simulink model "Track_green_simulation"  (R2021b)
settings: Solver=FixedStepDiscrete  StartTime=0.0  StopTime=inf  RelTol=1e-3  EnableMultiTasking=on
libraries: visionsinks x2, visiontextngfix x1, dspvision x1, simulink x1
settings Model: SimulationMode=external  ExtModeTrigDuration=100  Creator=edelaher  LastModifiedBy=litani
settings SolverCC: AlgebraicLoopSolver=TrustRegion  PositivePriorityOrder=on  AutoInsertRateTranBlk=on
settings DataIOCC: LimitDataPoints=on  SaveFormat=Array  ReturnWorkspaceOutputs=off
settings OptimizationCC: DefaultParameterBehavior=Inlined  MaxStackSize=64  EfficientTunableParamExpr=on
settings DebuggingCC: UnderspecifiedInitializationDetection=Classic  MergeDetectMultiDrivingBlocksExec=none  ParameterTunabilityLossMsg=error  AllowSymbolicDim=off  SFUnexpectedBacktrackingDiag=warning  SFNoUnconditionalDefaultTransitionDiag=warning  SFExecutionAtInitializationDiag=none  SFMachineParentedDataDiag=warning  ArithmeticOperatorsInVariantConditions=warning
settings HardwareCC: ProdBitPerPointer=32  ProdBitPerSizeT=32  ProdBitPerPtrDiffT=32  ProdLargestAtomicInteger=Long  ProdLargestAtomicFloat=Double  ProdWordSize=32  ProdHWDeviceType=ARM Compatible->ARM Cortex  UseEmbeddedCoderFeatures=off
settings ModelReferenceCC: PropagateSignalLabelsOutOfModel=off
settings SFSimCC: SimUseLocalCustomCode=off  MATLABDynamicMemAlloc=off  CustomCodeUndefinedFunction=UseInterfaceOnly
settings RTWCC: Description=Embedded Coder  SystemTargetFile=ert.tlc  TemplateMakefile=ert_default_tmf  GenerateReport=on  RTWVerbose=off  RTWUseLocalCustomCode=off  Toolchain=GNU GCC Embedded Linux  IncludeHyperlinkInReport=on  LaunchReport=on  GenerateTraceInfo=on  GenerateTraceReport=on  GenerateTraceReportSl=on  GenerateTraceReportSf=on  GenerateTraceReportEml=on
settings CodeAppCC: ForceParamTrailComments=on  IgnoreCustomStorageClasses=off  OperatorAnnotations=on  SimulinkDataObjDesc=on  SFDataObjDesc=on  MATLABFcnDesc=on  InsertBlockDesc=on  StateflowObjectComments=on  MATLABSourceComments=on
settings ERTTargetCC: MultiwordLength=2048  SupportNonInlinedSFcns=on  SupportVariableSizeSignals=on  ERTCustomFileTemplate=example_file_process.tlc
settings ConfigComp: CovMetricSettings=dw  CovSaveCumulativeToWorkspaceVar=on  CovSaveSingleToWorkspaceVar=on  CovExternalEMLEnable=off

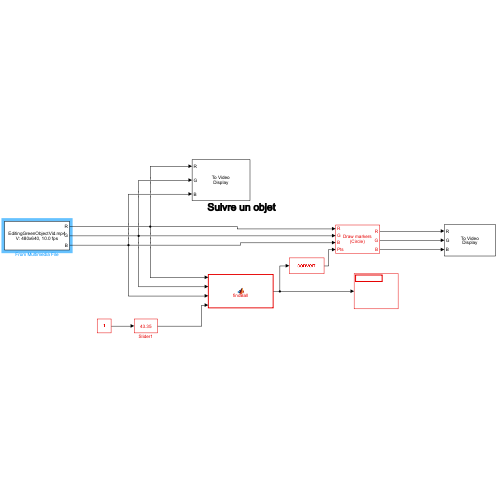
[thumbnail: Simulink's stored preview of the top-level diagram]
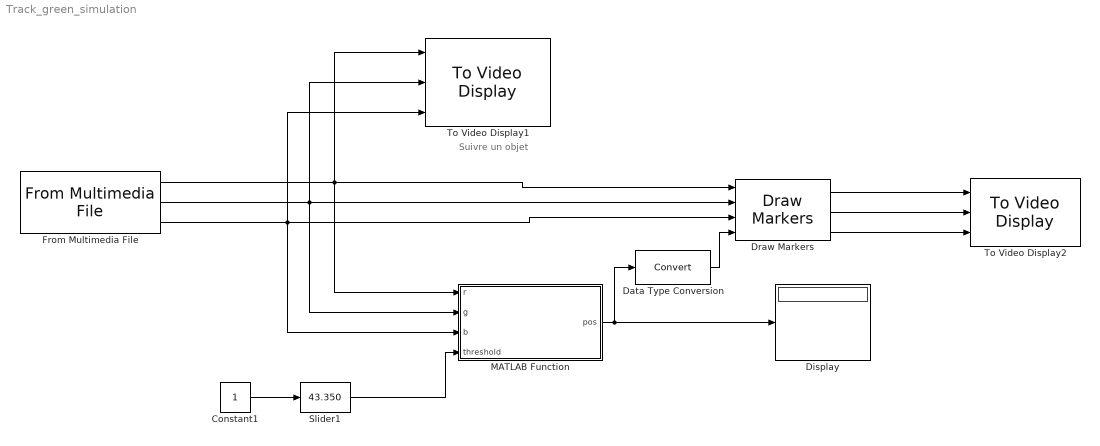
== system Track_green_simulation ==
  note: Suivre un objet
  Constant1 : Constant  OutDataTypeStr=uint8  SampleTime=0.1
  Data Type Conversion : DataTypeConversion
  Display : Display
  Draw Markers : visiontextngfix/Draw Markers  shape=Circle  size=3  fill=on  fillClrSource=Specify via dialog  display=User-specified value  intensity=200  color=[255 0 0]  opacity=1  viewport=Entire image  antialiasing=off  inType=Obsolete  imagePorts=Separate color signals  roundingMode=Floor  overflowMode=off
      settings: SourceProductBaseCode=VP
  From Multimedia File : dspvision/From Multimedia File  inputFilename=C:\Users\litani\OneDrive - MathWorks\Documents\Accounts overview\CentraleSupelec\Projects\TP ADAS_2020\HW\Mdl-and-presentation\Mdl\Instructor\EditingGreenObjectVid.mp4  readRange=[1 Inf]  loop=on  numPlays=inf  outputStreams=Video only  videoDataType=uint8  audioDataType=int16  inheritSampleTime=off  userDefinedSampleTime=0.1  noAudioOutput=off  isIntensityVideo=off  fourcc=RGB  colorVideoFormat=Separate color signals  outputEOF=off  dataOrg=Column-major  audioFrameSize=1024  computeAudioFrameSize=off  outSamplingMode=Sample based
  MATLAB Function : MATLAB Function  TreatAsAtomicUnit=on
  Slider1 : simulink/Math Operations/Slider Gain  gain=43.350  low=0  high=255
  To Video Display1 : visionsinks/To Video Display  windowSizeMode=Normal  openAtMdlStart=on  fullScreen=off  videoWindowX=127  videoWindowY=390  saveWindowSize=off  videoWindowWidth=640  videoWindowHeight=480  inputColorFormat=RGB  inputType=Obsolete  imagePorts=Separate color signals  OutputDevice=On-screen video monitor  dataOrg=Column-major  isWindowOpen=off
  To Video Display2 : visionsinks/To Video Display  windowSizeMode=Normal  openAtMdlStart=on  fullScreen=off  videoWindowX=770  videoWindowY=392  saveWindowSize=off  videoWindowWidth=640  videoWindowHeight=480  inputColorFormat=RGB  inputType=Obsolete  imagePorts=Separate color signals  OutputDevice=On-screen video monitor  dataOrg=Column-major  isWindowOpen=off
  wires:
  Draw Markers/1 -> To Video Display2/1
  MATLAB Function/1(pos) -> Data Type Conversion/1, Display/1
  Draw Markers/2 -> To Video Display2/2
  Draw Markers/3 -> To Video Display2/3
  Slider1/1 -> MATLAB Function/4(threshold)
  Constant1/1 -> Slider1/1
  Data Type Conversion/1 -> Draw Markers/4
  From Multimedia File/2 -> MATLAB Function/2(g), To Video Display1/2, Draw Markers/2
  From Multimedia File/3 -> To Video Display1/3, MATLAB Function/3(b), Draw Markers/3
  From Multimedia File/1 -> MATLAB Function/1(r), To Video Display1/1, Draw Markers/1

== matlab function Track_green_simulation/MATLAB Function ==
  data: r input; g input; b input; pos output; threshold input
function pos = findBall(r,g,b,threshold)
%#codegen
%% Calculate Green
% Then we perform an arithmetic operation on the matrices as a whole to try
% to create one matrix that represents an intensity of green.
justGreen = g - r/2 - b/2;

%% Threshold the image
% Now we can set a threshold to separate the parts of the image that we
% consider to be green from the rest.
bw = justGreen > threshold;

%% Find center
% Find the row and column location of the pixels and calculate the mean to get
% the approximate center of the ball.
[r,c] = find(bw);
if isempty(r)
    pos = [-1 -1];
else
    pos = [mean(c) mean(r)];
end
